simulink model "GS_model"  (R2018b)
settings: Solver=ode5  StartTime=0.0  StopTime=SimuStopTime  FixedStep=T_Simu  RelTol=1e-3
InitFcn:
  | Initial
undefined symbols (not defined in the file or in its folder): Aba10, Aba20, aeroCIP2006_S, aeroCIP2006_X, aeroCIP2006_Y, Agl0, Ass_kS, Ass_n1, Ass_n2, Ass_n3, Ass_n4, Ass_Noise, Ass_R, Ass_Resolution, Ass_TmOrder, AssA_Fix_Abs, AssB_Fix_Abs, AssC_Fix_Abs, AssD_Fix_Abs, AssE_Fix_Aps, AssF_Fix_Aps, C, c_max, c_min, Cd, CenterOfFigNX, CenterOfFigNY, CenterOfFigNZ, CenterOfFigP1, CenterOfFigP2, CenterOfFigPX, CenterOfFigPY, CenterOfFigPZ, Cmu, Crou, DEG2RAD, DiscIntNeverNeededParam, Eg_Dir, Eg_F, Eg_PrepareTime, Eg_r_L_L, Fw_Abf, Fw_Hmax, Fw_J, Fw_Spd0, Fw_Tmax, git_hash_BaseLine, git_hash_Project, Gnss_Noise_Pos, Gnss_Noise_Vel, Gnss_PropgationTime, GyroA_Fix_Abg, GyroA_Noise, GyroB_Fix_Abg, GyroB_Noise, GyroC_Fix_Abg, GyroC_Noise, GyroD_Fix_Abg, GyroD_Noise, h ... (+94)
libraries: simulink x308, sharedutil x46, aerolibutil x37, sharedtransform x31, vrlib x14, aerolibgravity2 x2
(part 9 of 20)

== system GS_model/Subsystem2/Subsystem/Sensor/StA&B&C&DModel1/StAMathModel3/StMathModel ==
  note: Qbs_St
  Qib : Inport
  Cons_StNoise : Inport  Port=2
  Qsb_StFix : Inport  Port=3
  TC_StFixErr : Inport  Port=4
  TC_StNoiseCoff : Inport  Port=5
  StNum : Inport  Port=6
  3 : Subsystem
  Constant : Constant  Value=0
  Constant1 : Constant  Value=0
  Demux : Demux  Outputs=[1;4]
  Demux1 : Demux  Outputs=2
  Logical Operator : Logic  Operator=OR  AllPortsSameDT=off  OutDataTypeStr=boolean
  Logical Operator1 : Logic  Operator=OR  AllPortsSameDT=off  OutDataTypeStr=boolean
  Quaternion Inverse : aerolibutil/Quaternion Inverse
  Quaternion Multiplication : aerolibutil/Quaternion Multiplication
  Quaternion Multiplication2 : aerolibutil/Quaternion Multiplication
  Quaternion Multiplication4 : aerolibutil/Quaternion Multiplication
  Quaternion Normalize : sharedutil/Quaternion Normalize  aMode=aMode
      settings: SourceProductBaseCode=AE,PW,MT,VE,VP
  Quaternion Normalize2 : sharedutil/Quaternion Normalize  aMode=aMode
      settings: SourceProductBaseCode=AE,PW,MT,VE,VP
  Relational Operator{,1..3} (4 alike) : RelationalOperator  Operator===  OutDataTypeStr=boolean  RndMeth=Simplest
  Triggered Subsystem1 : Subsystem  TreatAsAtomicUnit=on
  Triggered Subsystem2 : Subsystem  TreatAsAtomicUnit=on
  Qis_St : Outport
  wires:
  Quaternion Inverse/1 -> Quaternion Multiplication2/2
  Logical Operator1/1 -> Triggered Subsystem2/Enable
  Relational Operator3/1 -> Logical Operator1/1
  Constant1/1 -> Relational Operator3/1
  Relational Operator/1 -> Logical Operator1/2
  Logical Operator/1 -> Triggered Subsystem1/Enable
  Relational Operator2/1 -> Logical Operator/1
  Constant/1 -> Relational Operator2/1
  Relational Operator1/1 -> Logical Operator/2
  StNum/1 -> Relational Operator1/1, Relational Operator/1
  Cons_StNoise/1 -> 3/2(Cons_StNoise)
  Quaternion Multiplication4/1 -> Qis_St/1
  TC_StFixErr/1 -> Demux/1
  Qsb_StFix/1 -> Quaternion Normalize/1
  Qib/1 -> Quaternion Multiplication2/1
  Quaternion Multiplication/1 -> Quaternion Inverse/1
  3/1(Q_StNoise) -> Quaternion Multiplication4/2
  Quaternion Normalize2/1 -> Quaternion Multiplication/2
  TC_StNoiseCoff/1 -> Demux1/1
  Quaternion Multiplication2/1 -> Quaternion Multiplication4/1
  Demux/1 -> Relational Operator1/2, Relational Operator2/2
  Demux1/2 -> Triggered Subsystem2/1(In1)
  Demux1/1 -> Relational Operator/2, Relational Operator3/2
  Quaternion Normalize/1 -> Quaternion Multiplication/1
  Triggered Subsystem1/1(Out1) -> Quaternion Normalize2/1
  Demux/2 -> Triggered Subsystem1/1(In1)
  Triggered Subsystem2/1(Out1) -> 3/1(TC_StNoiseCoff)

== system GS_model/Subsystem2/Subsystem/Sensor/StA&B&C&DModel1/StAMathModel3/Subsystem ==
  note: 0-自主
      | 1-常有效
      | 2-常无效
  Sun_b : Inport
  Sunshine : Inport  Port=2
  Tc_ValidSet : Inport  Port=3
  Qsb_StAFix : Inport  Port=4
  SEA : Inport  Port=5
  EEA : Inport  Port=6
  Qob : Inport  Port=7
  Qis : Inport  Port=8
  StNum : Inport  Port=9
  Constant1 : Constant  Value=0
  Constant2 : Constant  Value=[1;0;0;0]
  Constant3 : Constant
  Constant4 : Constant  Value=0
  Demux1 : Demux  Outputs=2
  Logical Operator1 : Logic  Operator=OR  AllPortsSameDT=off  OutDataTypeStr=boolean
  Relational Operator : RelationalOperator  Operator===  OutDataTypeStr=boolean  RndMeth=Simplest
  Relational Operator3 : RelationalOperator  Operator===  OutDataTypeStr=boolean  RndMeth=Simplest
  Subsystem : Subsystem
  Switch : Switch  Criteria=u2 > Threshold  Threshold=0.5
  Switch1 : Switch  Criteria=u2 > Threshold  Threshold=0.5
  Switch2 : Switch  Criteria=u2 > Threshold  Threshold=1.5
  Triggered Subsystem2 : Subsystem  TreatAsAtomicUnit=on
  Agl_St&SunEarth : Outport
  Valid : Outport  Port=2
  Qis_St : Outport  Port=3
  wires:
  Constant2/1 -> Switch/3
  Qis/1 -> Switch/1
  Logical Operator1/1 -> Triggered Subsystem2/Enable
  Constant4/1 -> Switch2/1
  Switch1/1 -> Switch2/3
  Constant3/1 -> Switch1/1
  Subsystem/1(Valid) -> Switch1/3
  Triggered Subsystem2/1(Out1) -> Switch2/2, Switch1/2
  Tc_ValidSet/1 -> Demux1/1
  Demux1/1 -> Relational Operator/2, Relational Operator3/2
  StNum/1 -> Relational Operator/1
  Demux1/2 -> Triggered Subsystem2/1(In1)
  Constant1/1 -> Relational Operator3/1
  Relational Operator/1 -> Logical Operator1/2
  Relational Operator3/1 -> Logical Operator1/1
  Subsystem/2(Agl_St&SunEarth) -> Agl_St&SunEarth/1
  Qob/1 -> Subsystem/6(Qob)
  EEA/1 -> Subsystem/5(EEA)
  SEA/1 -> Subsystem/4(SEA)
  Qsb_StAFix/1 -> Subsystem/3(Qsb_StAFix)
  Sunshine/1 -> Subsystem/2(Sunshine)
  Sun_b/1 -> Subsystem/1(Sun_b)
  Switch2/1 -> Switch/2, Valid/1
  Switch/1 -> Qis_St/1

== system GS_model/Subsystem2/EquipmentCmd/Fw1/Subsystem7/Subsystem1/FWDataSourceChoice/CmdModeChoice ==
  note: UDP指令来源：复用星上链路标志，默认AA
      | AA -- FC指令
      | 55 -- 直接指令
  note: 动力学链路，默认0
      | 1 -- 422
      | 0 -- UDP
  FW_Data_Source : Inport
  FW_CmdMode : Inport  Port=2
  422 : Subsystem  TreatAsAtomicUnit=on
  Demux : Demux  Outputs=2
  FC : Subsystem  TreatAsAtomicUnit=on
  If : If  NumInputs=2  IfExpression=u1 > 0.5  ElseIfExpressions=u1<0.5 & u2<100
  Merge : Merge  Inputs=3
  Selector : Selector  InputPortWidth=3  IndexOptions=Index vector (dialog)  Indices=1  OutputSizes=1
  Selector1 : Selector  InputPortWidth=3  IndexOptions=Index vector (dialog)  Indices=2  OutputSizes=1
  Selector2 : Selector  InputPortWidth=3  IndexOptions=Index vector (dialog)  Indices=3  OutputSizes=1
  UDP : Subsystem  TreatAsAtomicUnit=on
  FW_Cmd_Mode : Outport
  wires:
  Demux/2 -> If/2
  If/3 -> FC/Action
  If/2 -> UDP/Action
  If/1 -> 422/Action
  FW_Data_Source/1 -> Demux/1
  Demux/1 -> If/1
  Selector2/1 -> FC/1(In1)
  Selector1/1 -> UDP/1(In1)
  Selector/1 -> 422/1(In1)
  Merge/1 -> FW_Cmd_Mode/1
  FC/1(Out1) -> Merge/3
  UDP/1(Out1) -> Merge/2
  422/1(Out1) -> Merge/1
  FW_CmdMode/1 -> Selector/1, Selector1/1, Selector2/1

== system GS_model/Subsystem2/EquipmentCmd/Fw1/Subsystem7/Subsystem1/FWDataSourceChoice/CmdSpdChoice ==
  note: Fc_DataSource      Tc_DataSource
      | AA-真采集（默认）  1-422(DB9);
      |                                  0-反测（默认
      | 55 -伪采集                UDP
  note: AA -- FC
      | 55 -- udp
  note: 1 -- 422
      | 0 -- else
  note: Fc_DataSource
  note: Tc_DataSource
  FW_Data_Source : Inport
  FW_CmdSpd : Inport  Port=2
  422 : Subsystem  TreatAsAtomicUnit=on
  Demux : Demux  Outputs=2
  FC : Subsystem  TreatAsAtomicUnit=on
  If : If  NumInputs=2  IfExpression=u1 > 0.5  ElseIfExpressions=u1<0.5 & u2<100
  Merge : Merge  Inputs=3
  Selector : Selector  InputPortWidth=3  IndexOptions=Index vector (dialog)  Indices=1  OutputSizes=1
  Selector1 : Selector  InputPortWidth=3  IndexOptions=Index vector (dialog)  Indices=2  OutputSizes=1
  Selector2 : Selector  InputPortWidth=3  IndexOptions=Index vector (dialog)  Indices=3  OutputSizes=1
  UDP : Subsystem  TreatAsAtomicUnit=on
  FW_Cmd_Spd : Outport
  wires:
  Demux/2 -> If/2
  If/3 -> FC/Action
  If/2 -> UDP/Action
  If/1 -> 422/Action
  FW_Data_Source/1 -> Demux/1
  Demux/1 -> If/1
  Selector2/1 -> FC/1(In1)
  Selector1/1 -> UDP/1(In1)
  Selector/1 -> 422/1(In1)
  Merge/1 -> FW_Cmd_Spd/1
  FC/1(Out1) -> Merge/3
  UDP/1(Out1) -> Merge/2
  422/1(Out1) -> Merge/1
  FW_CmdSpd/1 -> Selector/1, Selector1/1, Selector2/1

== system GS_model/Subsystem2/EquipmentCmd/Fw1/Subsystem7/Subsystem1/FWDataSourceChoice/CmdTChoice ==
  note: 1 -- 422
      | 0 -- else
  note: AA -- FC
      | 55 -- udp
  FW_Data_Source : Inport
  FW_CmdTorque : Inport  Port=2
  422 : Subsystem  TreatAsAtomicUnit=on
  Demux : Demux  Outputs=2
  FC : Subsystem  TreatAsAtomicUnit=on
  If : If  NumInputs=2  IfExpression=u1 > 0.5  ElseIfExpressions=u1<0.5 & u2<100
  Merge : Merge  Inputs=3
  Selector : Selector  InputPortWidth=3  IndexOptions=Index vector (dialog)  Indices=1  OutputSizes=1
  Selector1 : Selector  InputPortWidth=3  IndexOptions=Index vector (dialog)  Indices=2  OutputSizes=1
  Selector2 : Selector  InputPortWidth=3  IndexOptions=Index vector (dialog)  Indices=3  OutputSizes=1
  UDP : Subsystem  TreatAsAtomicUnit=on
  FW_Cmd_T : Outport
  wires:
  FW_CmdTorque/1 -> Selector2/1, Selector1/1, Selector/1
  422/1(Out1) -> Merge/1
  UDP/1(Out1) -> Merge/2
  FC/1(Out1) -> Merge/3
  Merge/1 -> FW_Cmd_T/1
  Selector/1 -> 422/1(In1)
  Selector1/1 -> UDP/1(In1)
  Selector2/1 -> FC/1(In1)
  Demux/1 -> If/1
  FW_Data_Source/1 -> Demux/1
  If/1 -> 422/Action
  If/2 -> UDP/Action
  If/3 -> FC/Action
  Demux/2 -> If/2

== system GS_model/Subsystem2/EquipmentCmd/Fw1/Subsystem7/Subsystem2/FWDataSourceChoice/CmdModeChoice ==
  note: 动力学链路，默认0
      | 1 -- 422
      | 0 -- UDP
  note: UDP指令来源：复用星上链路标志，默认AA
      | AA -- FC指令
      | 55 -- 直接指令
  FW_Data_Source : Inport
  FW_CmdMode : Inport  Port=2
  422 : Subsystem  TreatAsAtomicUnit=on
  Demux : Demux  Outputs=2
  FC : Subsystem  TreatAsAtomicUnit=on
  If : If  NumInputs=2  IfExpression=u1 > 0.5  ElseIfExpressions=u1<0.5 & u2<100
  Merge : Merge  Inputs=3
  Selector : Selector  InputPortWidth=3  IndexOptions=Index vector (dialog)  Indices=1  OutputSizes=1
  Selector1 : Selector  InputPortWidth=3  IndexOptions=Index vector (dialog)  Indices=2  OutputSizes=1
  Selector2 : Selector  InputPortWidth=3  IndexOptions=Index vector (dialog)  Indices=3  OutputSizes=1
  UDP : Subsystem  TreatAsAtomicUnit=on
  FW_Cmd_Mode : Outport
  wires:
  FW_CmdMode/1 -> Selector2/1, Selector1/1, Selector/1
  422/1(Out1) -> Merge/1
  UDP/1(Out1) -> Merge/2
  FC/1(Out1) -> Merge/3
  Merge/1 -> FW_Cmd_Mode/1
  Selector/1 -> 422/1(In1)
  Selector1/1 -> UDP/1(In1)
  Selector2/1 -> FC/1(In1)
  Demux/1 -> If/1
  FW_Data_Source/1 -> Demux/1
  If/1 -> 422/Action
  If/2 -> UDP/Action
  If/3 -> FC/Action
  Demux/2 -> If/2

== system GS_model/Subsystem2/EquipmentCmd/Fw1/Subsystem7/Subsystem2/FWDataSourceChoice/CmdSpdChoice ==
  note: Tc_DataSource
  note: Fc_DataSource
  note: 1 -- 422
      | 0 -- else
  note: AA -- FC
      | 55 -- udp
  note: Fc_DataSource      Tc_DataSource
      | AA-真采集（默认）  1-422(DB9);
      |                                  0-反测（默认
      | 55 -伪采集                UDP
  FW_Data_Source : Inport
  FW_CmdSpd : Inport  Port=2
  422 : Subsystem  TreatAsAtomicUnit=on
  Demux : Demux  Outputs=2
  FC : Subsystem  TreatAsAtomicUnit=on
  If : If  NumInputs=2  IfExpression=u1 > 0.5  ElseIfExpressions=u1<0.5 & u2<100
  Merge : Merge  Inputs=3
  Selector : Selector  InputPortWidth=3  IndexOptions=Index vector (dialog)  Indices=1  OutputSizes=1
  Selector1 : Selector  InputPortWidth=3  IndexOptions=Index vector (dialog)  Indices=2  OutputSizes=1
  Selector2 : Selector  InputPortWidth=3  IndexOptions=Index vector (dialog)  Indices=3  OutputSizes=1
  UDP : Subsystem  TreatAsAtomicUnit=on
  FW_Cmd_Spd : Outport
  wires:
  FW_CmdSpd/1 -> Selector2/1, Selector1/1, Selector/1
  422/1(Out1) -> Merge/1
  UDP/1(Out1) -> Merge/2
  FC/1(Out1) -> Merge/3
  Merge/1 -> FW_Cmd_Spd/1
  Selector/1 -> 422/1(In1)
  Selector1/1 -> UDP/1(In1)
  Selector2/1 -> FC/1(In1)
  Demux/1 -> If/1
  FW_Data_Source/1 -> Demux/1
  If/1 -> 422/Action
  If/2 -> UDP/Action
  If/3 -> FC/Action
  Demux/2 -> If/2

== system GS_model/Subsystem2/EquipmentCmd/Fw1/Subsystem7/Subsystem2/FWDataSourceChoice/CmdTChoice ==
  note: AA -- FC
      | 55 -- udp
  note: 1 -- 422
      | 0 -- else
  FW_Data_Source : Inport
  FW_CmdTorque : Inport  Port=2
  422 : Subsystem  TreatAsAtomicUnit=on
  Demux : Demux  Outputs=2
  FC : Subsystem  TreatAsAtomicUnit=on
  If : If  NumInputs=2  IfExpression=u1 > 0.5  ElseIfExpressions=u1<0.5 & u2<100
  Merge : Merge  Inputs=3
  Selector : Selector  InputPortWidth=3  IndexOptions=Index vector (dialog)  Indices=1  OutputSizes=1
  Selector1 : Selector  InputPortWidth=3  IndexOptions=Index vector (dialog)  Indices=2  OutputSizes=1
  Selector2 : Selector  InputPortWidth=3  IndexOptions=Index vector (dialog)  Indices=3  OutputSizes=1
  UDP : Subsystem  TreatAsAtomicUnit=on
  FW_Cmd_T : Outport
  wires:
  Demux/2 -> If/2
  If/3 -> FC/Action
  If/2 -> UDP/Action
  If/1 -> 422/Action
  FW_Data_Source/1 -> Demux/1
  Demux/1 -> If/1
  Selector2/1 -> FC/1(In1)
  Selector1/1 -> UDP/1(In1)
  Selector/1 -> 422/1(In1)
  Merge/1 -> FW_Cmd_T/1
  FC/1(Out1) -> Merge/3
  UDP/1(Out1) -> Merge/2
  422/1(Out1) -> Merge/1
  FW_CmdTorque/1 -> Selector/1, Selector1/1, Selector2/1

== system GS_model/Subsystem2/EquipmentCmd/Fw1/Subsystem7/Subsystem3/FWDataSourceChoice/CmdModeChoice ==
  note: UDP指令来源：复用星上链路标志，默认AA
      | AA -- FC指令
      | 55 -- 直接指令
  note: 动力学链路，默认0
      | 1 -- 422
      | 0 -- UDP
  FW_Data_Source : Inport
  FW_CmdMode : Inport  Port=2
  422 : Subsystem  TreatAsAtomicUnit=on
  Demux : Demux  Outputs=2
  FC : Subsystem  TreatAsAtomicUnit=on
  If : If  NumInputs=2  IfExpression=u1 > 0.5  ElseIfExpressions=u1<0.5 & u2<100
  Merge : Merge  Inputs=3
  Selector : Selector  InputPortWidth=3  IndexOptions=Index vector (dialog)  Indices=1  OutputSizes=1
  Selector1 : Selector  InputPortWidth=3  IndexOptions=Index vector (dialog)  Indices=2  OutputSizes=1
  Selector2 : Selector  InputPortWidth=3  IndexOptions=Index vector (dialog)  Indices=3  OutputSizes=1
  UDP : Subsystem  TreatAsAtomicUnit=on
  FW_Cmd_Mode : Outport
  wires:
  Demux/2 -> If/2
  If/3 -> FC/Action
  If/2 -> UDP/Action
  If/1 -> 422/Action
  FW_Data_Source/1 -> Demux/1
  Demux/1 -> If/1
  Selector2/1 -> FC/1(In1)
  Selector1/1 -> UDP/1(In1)
  Selector/1 -> 422/1(In1)
  Merge/1 -> FW_Cmd_Mode/1
  FC/1(Out1) -> Merge/3
  UDP/1(Out1) -> Merge/2
  422/1(Out1) -> Merge/1
  FW_CmdMode/1 -> Selector/1, Selector1/1, Selector2/1

== system GS_model/Subsystem2/EquipmentCmd/Fw1/Subsystem7/Subsystem3/FWDataSourceChoice/CmdSpdChoice ==
  note: Fc_DataSource      Tc_DataSource
      | AA-真采集（默认）  1-422(DB9);
      |                                  0-反测（默认
      | 55 -伪采集                UDP
  note: AA -- FC
      | 55 -- udp
  note: 1 -- 422
      | 0 -- else
  note: Fc_DataSource
  note: Tc_DataSource
  FW_Data_Source : Inport
  FW_CmdSpd : Inport  Port=2
  422 : Subsystem  TreatAsAtomicUnit=on
  Demux : Demux  Outputs=2
  FC : Subsystem  TreatAsAtomicUnit=on
  If : If  NumInputs=2  IfExpression=u1 > 0.5  ElseIfExpressions=u1<0.5 & u2<100
  Merge : Merge  Inputs=3
  Selector : Selector  InputPortWidth=3  IndexOptions=Index vector (dialog)  Indices=1  OutputSizes=1
  Selector1 : Selector  InputPortWidth=3  IndexOptions=Index vector (dialog)  Indices=2  OutputSizes=1
  Selector2 : Selector  InputPortWidth=3  IndexOptions=Index vector (dialog)  Indices=3  OutputSizes=1
  UDP : Subsystem  TreatAsAtomicUnit=on
  FW_Cmd_Spd : Outport
  wires:
  Demux/2 -> If/2
  If/3 -> FC/Action
  If/2 -> UDP/Action
  If/1 -> 422/Action
  FW_Data_Source/1 -> Demux/1
  Demux/1 -> If/1
  Selector2/1 -> FC/1(In1)
  Selector1/1 -> UDP/1(In1)
  Selector/1 -> 422/1(In1)
  Merge/1 -> FW_Cmd_Spd/1
  FC/1(Out1) -> Merge/3
  UDP/1(Out1) -> Merge/2
  422/1(Out1) -> Merge/1
  FW_CmdSpd/1 -> Selector/1, Selector1/1, Selector2/1

== system GS_model/Subsystem2/EquipmentCmd/Fw1/Subsystem7/Subsystem3/FWDataSourceChoice/CmdTChoice ==
  note: 1 -- 422
      | 0 -- else
  note: AA -- FC
      | 55 -- udp
  FW_Data_Source : Inport
  FW_CmdTorque : Inport  Port=2
  422 : Subsystem  TreatAsAtomicUnit=on
  Demux : Demux  Outputs=2
  FC : Subsystem  TreatAsAtomicUnit=on
  If : If  NumInputs=2  IfExpression=u1 > 0.5  ElseIfExpressions=u1<0.5 & u2<100
  Merge : Merge  Inputs=3
  Selector : Selector  InputPortWidth=3  IndexOptions=Index vector (dialog)  Indices=1  OutputSizes=1
  Selector1 : Selector  InputPortWidth=3  IndexOptions=Index vector (dialog)  Indices=2  OutputSizes=1
  Selector2 : Selector  InputPortWidth=3  IndexOptions=Index vector (dialog)  Indices=3  OutputSizes=1
  UDP : Subsystem  TreatAsAtomicUnit=on
  FW_Cmd_T : Outport
  wires:
  FW_CmdTorque/1 -> Selector2/1, Selector1/1, Selector/1
  422/1(Out1) -> Merge/1
  UDP/1(Out1) -> Merge/2
  FC/1(Out1) -> Merge/3
  Merge/1 -> FW_Cmd_T/1
  Selector/1 -> 422/1(In1)
  Selector1/1 -> UDP/1(In1)
  Selector2/1 -> FC/1(In1)
  Demux/1 -> If/1
  FW_Data_Source/1 -> Demux/1
  If/1 -> 422/Action
  If/2 -> UDP/Action
  If/3 -> FC/Action
  Demux/2 -> If/2

== system GS_model/Subsystem2/EquipmentCmd/Fw1/Subsystem7/Subsystem4/FWDataSourceChoice/CmdModeChoice ==
  note: 动力学链路，默认0
      | 1 -- 422
      | 0 -- UDP
  note: UDP指令来源：复用星上链路标志，默认AA
      | AA -- FC指令
      | 55 -- 直接指令
  FW_Data_Source : Inport
  FW_CmdMode : Inport  Port=2
  422 : Subsystem  TreatAsAtomicUnit=on
  Demux : Demux  Outputs=2
  FC : Subsystem  TreatAsAtomicUnit=on
  If : If  NumInputs=2  IfExpression=u1 > 0.5  ElseIfExpressions=u1<0.5 & u2<100
  Merge : Merge  Inputs=3
  Selector : Selector  InputPortWidth=3  IndexOptions=Index vector (dialog)  Indices=1  OutputSizes=1
  Selector1 : Selector  InputPortWidth=3  IndexOptions=Index vector (dialog)  Indices=2  OutputSizes=1
  Selector2 : Selector  InputPortWidth=3  IndexOptions=Index vector (dialog)  Indices=3  OutputSizes=1
  UDP : Subsystem  TreatAsAtomicUnit=on
  FW_Cmd_Mode : Outport
  wires:
  FW_CmdMode/1 -> Selector2/1, Selector1/1, Selector/1
  422/1(Out1) -> Merge/1
  UDP/1(Out1) -> Merge/2
  FC/1(Out1) -> Merge/3
  Merge/1 -> FW_Cmd_Mode/1
  Selector/1 -> 422/1(In1)
  Selector1/1 -> UDP/1(In1)
  Selector2/1 -> FC/1(In1)
  Demux/1 -> If/1
  FW_Data_Source/1 -> Demux/1
  If/1 -> 422/Action
  If/2 -> UDP/Action
  If/3 -> FC/Action
  Demux/2 -> If/2

== system GS_model/Subsystem2/EquipmentCmd/Fw1/Subsystem7/Subsystem4/FWDataSourceChoice/CmdSpdChoice ==
  note: Tc_DataSource
  note: Fc_DataSource
  note: 1 -- 422
      | 0 -- else
  note: AA -- FC
      | 55 -- udp
  note: Fc_DataSource      Tc_DataSource
      | AA-真采集（默认）  1-422(DB9);
      |                                  0-反测（默认
      | 55 -伪采集                UDP
  FW_Data_Source : Inport
  FW_CmdSpd : Inport  Port=2
  422 : Subsystem  TreatAsAtomicUnit=on
  Demux : Demux  Outputs=2
  FC : Subsystem  TreatAsAtomicUnit=on
  If : If  NumInputs=2  IfExpression=u1 > 0.5  ElseIfExpressions=u1<0.5 & u2<100
  Merge : Merge  Inputs=3
  Selector : Selector  InputPortWidth=3  IndexOptions=Index vector (dialog)  Indices=1  OutputSizes=1
  Selector1 : Selector  InputPortWidth=3  IndexOptions=Index vector (dialog)  Indices=2  OutputSizes=1
  Selector2 : Selector  InputPortWidth=3  IndexOptions=Index vector (dialog)  Indices=3  OutputSizes=1
  UDP : Subsystem  TreatAsAtomicUnit=on
  FW_Cmd_Spd : Outport
  wires:
  FW_CmdSpd/1 -> Selector2/1, Selector1/1, Selector/1
  422/1(Out1) -> Merge/1
  UDP/1(Out1) -> Merge/2
  FC/1(Out1) -> Merge/3
  Merge/1 -> FW_Cmd_Spd/1
  Selector/1 -> 422/1(In1)
  Selector1/1 -> UDP/1(In1)
  Selector2/1 -> FC/1(In1)
  Demux/1 -> If/1
  FW_Data_Source/1 -> Demux/1
  If/1 -> 422/Action
  If/2 -> UDP/Action
  If/3 -> FC/Action
  Demux/2 -> If/2

== system GS_model/Subsystem2/EquipmentCmd/Fw1/Subsystem7/Subsystem4/FWDataSourceChoice/CmdTChoice ==
  note: AA -- FC
      | 55 -- udp
  note: 1 -- 422
      | 0 -- else
  FW_Data_Source : Inport
  FW_CmdTorque : Inport  Port=2
  422 : Subsystem  TreatAsAtomicUnit=on
  Demux : Demux  Outputs=2
  FC : Subsystem  TreatAsAtomicUnit=on
  If : If  NumInputs=2  IfExpression=u1 > 0.5  ElseIfExpressions=u1<0.5 & u2<100
  Merge : Merge  Inputs=3
  Selector : Selector  InputPortWidth=3  IndexOptions=Index vector (dialog)  Indices=1  OutputSizes=1
  Selector1 : Selector  InputPortWidth=3  IndexOptions=Index vector (dialog)  Indices=2  OutputSizes=1
  Selector2 : Selector  InputPortWidth=3  IndexOptions=Index vector (dialog)  Indices=3  OutputSizes=1
  UDP : Subsystem  TreatAsAtomicUnit=on
  FW_Cmd_T : Outport
  wires:
  Demux/2 -> If/2
  If/3 -> FC/Action
  If/2 -> UDP/Action
  If/1 -> 422/Action
  FW_Data_Source/1 -> Demux/1
  Demux/1 -> If/1
  Selector2/1 -> FC/1(In1)
  Selector1/1 -> UDP/1(In1)
  Selector/1 -> 422/1(In1)
  Merge/1 -> FW_Cmd_T/1
  FC/1(Out1) -> Merge/3
  UDP/1(Out1) -> Merge/2
  422/1(Out1) -> Merge/1
  FW_CmdTorque/1 -> Selector/1, Selector1/1, Selector2/1

== system GS_model/Subsystem2/EquipmentCmd/Fw1/Subsystem7/Subsystem5/FWDataSourceChoice/CmdModeChoice ==
  note: UDP指令来源：复用星上链路标志，默认AA
      | AA -- FC指令
      | 55 -- 直接指令
  note: 动力学链路，默认0
      | 1 -- 422
      | 0 -- UDP
  FW_Data_Source : Inport
  FW_CmdMode : Inport  Port=2
  422 : Subsystem  TreatAsAtomicUnit=on
  Demux : Demux  Outputs=2
  FC : Subsystem  TreatAsAtomicUnit=on
  If : If  NumInputs=2  IfExpression=u1 > 0.5  ElseIfExpressions=u1<0.5 & u2<100
  Merge : Merge  Inputs=3
  Selector : Selector  InputPortWidth=3  IndexOptions=Index vector (dialog)  Indices=1  OutputSizes=1
  Selector1 : Selector  InputPortWidth=3  IndexOptions=Index vector (dialog)  Indices=2  OutputSizes=1
  Selector2 : Selector  InputPortWidth=3  IndexOptions=Index vector (dialog)  Indices=3  OutputSizes=1
  UDP : Subsystem  TreatAsAtomicUnit=on
  FW_Cmd_Mode : Outport
  wires:
  Demux/2 -> If/2
  If/3 -> FC/Action
  If/2 -> UDP/Action
  If/1 -> 422/Action
  FW_Data_Source/1 -> Demux/1
  Demux/1 -> If/1
  Selector2/1 -> FC/1(In1)
  Selector1/1 -> UDP/1(In1)
  Selector/1 -> 422/1(In1)
  Merge/1 -> FW_Cmd_Mode/1
  FC/1(Out1) -> Merge/3
  UDP/1(Out1) -> Merge/2
  422/1(Out1) -> Merge/1
  FW_CmdMode/1 -> Selector/1, Selector1/1, Selector2/1

== system GS_model/Subsystem2/EquipmentCmd/Fw1/Subsystem7/Subsystem5/FWDataSourceChoice/CmdSpdChoice ==
  note: Fc_DataSource      Tc_DataSource
      | AA-真采集（默认）  1-422(DB9);
      |                                  0-反测（默认
      | 55 -伪采集                UDP
  note: AA -- FC
      | 55 -- udp
  note: 1 -- 422
      | 0 -- else
  note: Fc_DataSource
  note: Tc_DataSource
  FW_Data_Source : Inport
  FW_CmdSpd : Inport  Port=2
  422 : Subsystem  TreatAsAtomicUnit=on
  Demux : Demux  Outputs=2
  FC : Subsystem  TreatAsAtomicUnit=on
  If : If  NumInputs=2  IfExpression=u1 > 0.5  ElseIfExpressions=u1<0.5 & u2<100
  Merge : Merge  Inputs=3
  Selector : Selector  InputPortWidth=3  IndexOptions=Index vector (dialog)  Indices=1  OutputSizes=1
  Selector1 : Selector  InputPortWidth=3  IndexOptions=Index vector (dialog)  Indices=2  OutputSizes=1
  Selector2 : Selector  InputPortWidth=3  IndexOptions=Index vector (dialog)  Indices=3  OutputSizes=1
  UDP : Subsystem  TreatAsAtomicUnit=on
  FW_Cmd_Spd : Outport
  wires:
  Demux/2 -> If/2
  If/3 -> FC/Action
  If/2 -> UDP/Action
  If/1 -> 422/Action
  FW_Data_Source/1 -> Demux/1
  Demux/1 -> If/1
  Selector2/1 -> FC/1(In1)
  Selector1/1 -> UDP/1(In1)
  Selector/1 -> 422/1(In1)
  Merge/1 -> FW_Cmd_Spd/1
  FC/1(Out1) -> Merge/3
  UDP/1(Out1) -> Merge/2
  422/1(Out1) -> Merge/1
  FW_CmdSpd/1 -> Selector/1, Selector1/1, Selector2/1

== system GS_model/Subsystem2/EquipmentCmd/Fw1/Subsystem7/Subsystem5/FWDataSourceChoice/CmdTChoice ==
  note: 1 -- 422
      | 0 -- else
  note: AA -- FC
      | 55 -- udp
  FW_Data_Source : Inport
  FW_CmdTorque : Inport  Port=2
  422 : Subsystem  TreatAsAtomicUnit=on
  Demux : Demux  Outputs=2
  FC : Subsystem  TreatAsAtomicUnit=on
  If : If  NumInputs=2  IfExpression=u1 > 0.5  ElseIfExpressions=u1<0.5 & u2<100
  Merge : Merge  Inputs=3
  Selector : Selector  InputPortWidth=3  IndexOptions=Index vector (dialog)  Indices=1  OutputSizes=1
  Selector1 : Selector  InputPortWidth=3  IndexOptions=Index vector (dialog)  Indices=2  OutputSizes=1
  Selector2 : Selector  InputPortWidth=3  IndexOptions=Index vector (dialog)  Indices=3  OutputSizes=1
  UDP : Subsystem  TreatAsAtomicUnit=on
  FW_Cmd_T : Outport
  wires:
  FW_CmdTorque/1 -> Selector2/1, Selector1/1, Selector/1
  422/1(Out1) -> Merge/1
  UDP/1(Out1) -> Merge/2
  FC/1(Out1) -> Merge/3
  Merge/1 -> FW_Cmd_T/1
  Selector/1 -> 422/1(In1)
  Selector1/1 -> UDP/1(In1)
  Selector2/1 -> FC/1(In1)
  Demux/1 -> If/1
  FW_Data_Source/1 -> Demux/1
  If/1 -> 422/Action
  If/2 -> UDP/Action
  If/3 -> FC/Action
  Demux/2 -> If/2

== system GS_model/Subsystem2/EquipmentCmd/Fw1/Subsystem7/Subsystem6/FWDataSourceChoice/CmdModeChoice ==
  note: 动力学链路，默认0
      | 1 -- 422
      | 0 -- UDP
  note: UDP指令来源：复用星上链路标志，默认AA
      | AA -- FC指令
      | 55 -- 直接指令
  FW_Data_Source : Inport
  FW_CmdMode : Inport  Port=2
  422 : Subsystem  TreatAsAtomicUnit=on
  Demux : Demux  Outputs=2
  FC : Subsystem  TreatAsAtomicUnit=on
  If : If  NumInputs=2  IfExpression=u1 > 0.5  ElseIfExpressions=u1<0.5 & u2<100
  Merge : Merge  Inputs=3
  Selector : Selector  InputPortWidth=3  IndexOptions=Index vector (dialog)  Indices=1  OutputSizes=1
  Selector1 : Selector  InputPortWidth=3  IndexOptions=Index vector (dialog)  Indices=2  OutputSizes=1
  Selector2 : Selector  InputPortWidth=3  IndexOptions=Index vector (dialog)  Indices=3  OutputSizes=1
  UDP : Subsystem  TreatAsAtomicUnit=on
  FW_Cmd_Mode : Outport
  wires:
  FW_CmdMode/1 -> Selector2/1, Selector1/1, Selector/1
  422/1(Out1) -> Merge/1
  UDP/1(Out1) -> Merge/2
  FC/1(Out1) -> Merge/3
  Merge/1 -> FW_Cmd_Mode/1
  Selector/1 -> 422/1(In1)
  Selector1/1 -> UDP/1(In1)
  Selector2/1 -> FC/1(In1)
  Demux/1 -> If/1
  FW_Data_Source/1 -> Demux/1
  If/1 -> 422/Action
  If/2 -> UDP/Action
  If/3 -> FC/Action
  Demux/2 -> If/2

== system GS_model/Subsystem2/EquipmentCmd/Fw1/Subsystem7/Subsystem6/FWDataSourceChoice/CmdSpdChoice ==
  note: Tc_DataSource
  note: Fc_DataSource
  note: 1 -- 422
      | 0 -- else
  note: AA -- FC
      | 55 -- udp
  note: Fc_DataSource      Tc_DataSource
      | AA-真采集（默认）  1-422(DB9);
      |                                  0-反测（默认
      | 55 -伪采集                UDP
  FW_Data_Source : Inport
  FW_CmdSpd : Inport  Port=2
  422 : Subsystem  TreatAsAtomicUnit=on
  Demux : Demux  Outputs=2
  FC : Subsystem  TreatAsAtomicUnit=on
  If : If  NumInputs=2  IfExpression=u1 > 0.5  ElseIfExpressions=u1<0.5 & u2<100
  Merge : Merge  Inputs=3
  Selector : Selector  InputPortWidth=3  IndexOptions=Index vector (dialog)  Indices=1  OutputSizes=1
  Selector1 : Selector  InputPortWidth=3  IndexOptions=Index vector (dialog)  Indices=2  OutputSizes=1
  Selector2 : Selector  InputPortWidth=3  IndexOptions=Index vector (dialog)  Indices=3  OutputSizes=1
  UDP : Subsystem  TreatAsAtomicUnit=on
  FW_Cmd_Spd : Outport
  wires:
  FW_CmdSpd/1 -> Selector2/1, Selector1/1, Selector/1
  422/1(Out1) -> Merge/1
  UDP/1(Out1) -> Merge/2
  FC/1(Out1) -> Merge/3
  Merge/1 -> FW_Cmd_Spd/1
  Selector/1 -> 422/1(In1)
  Selector1/1 -> UDP/1(In1)
  Selector2/1 -> FC/1(In1)
  Demux/1 -> If/1
  FW_Data_Source/1 -> Demux/1
  If/1 -> 422/Action
  If/2 -> UDP/Action
  If/3 -> FC/Action
  Demux/2 -> If/2

== system GS_model/Subsystem2/EquipmentCmd/Fw1/Subsystem7/Subsystem6/FWDataSourceChoice/CmdTChoice ==
  note: AA -- FC
      | 55 -- udp
  note: 1 -- 422
      | 0 -- else
  FW_Data_Source : Inport
  FW_CmdTorque : Inport  Port=2
  422 : Subsystem  TreatAsAtomicUnit=on
  Demux : Demux  Outputs=2
  FC : Subsystem  TreatAsAtomicUnit=on
  If : If  NumInputs=2  IfExpression=u1 > 0.5  ElseIfExpressions=u1<0.5 & u2<100
  Merge : Merge  Inputs=3
  Selector : Selector  InputPortWidth=3  IndexOptions=Index vector (dialog)  Indices=1  OutputSizes=1
  Selector1 : Selector  InputPortWidth=3  IndexOptions=Index vector (dialog)  Indices=2  OutputSizes=1
  Selector2 : Selector  InputPortWidth=3  IndexOptions=Index vector (dialog)  Indices=3  OutputSizes=1
  UDP : Subsystem  TreatAsAtomicUnit=on
  FW_Cmd_T : Outport
  wires:
  Demux/2 -> If/2
  If/3 -> FC/Action
  If/2 -> UDP/Action
  If/1 -> 422/Action
  FW_Data_Source/1 -> Demux/1
  Demux/1 -> If/1
  Selector2/1 -> FC/1(In1)
  Selector1/1 -> UDP/1(In1)
  Selector/1 -> 422/1(In1)
  Merge/1 -> FW_Cmd_T/1
  FC/1(Out1) -> Merge/3
  UDP/1(Out1) -> Merge/2
  422/1(Out1) -> Merge/1
  FW_CmdTorque/1 -> Selector/1, Selector1/1, Selector2/1

== system GS_model/Subsystem2/Subsystem/Actuator/Engine/Subsystem/Subsystem/Triggered Subsystem1 ==
  In1 : Inport
  Enable : EnablePort
  Out1 : Outport  InitialOutput=0
  wires:
  In1/1 -> Out1/1

== system GS_model/Subsystem2/Subsystem/Actuator/Engine/Subsystem/Subsystem1/Triggered Subsystem1 ==
  In1 : Inport
  Enable : EnablePort
  Out1 : Outport  InitialOutput=0
  wires:
  In1/1 -> Out1/1

== system GS_model/Subsystem2/Subsystem/Actuator/Engine/Subsystem/Subsystem2/Triggered Subsystem1 ==
  In1 : Inport
  Enable : EnablePort
  Out1 : Outport  InitialOutput=0
  wires:
  In1/1 -> Out1/1

== system GS_model/Subsystem2/Subsystem/Actuator/Engine/Subsystem1/Subsystem/Triggered Subsystem1 ==
  In1 : Inport
  Enable : EnablePort
  Out1 : Outport  InitialOutput=0
  wires:
  In1/1 -> Out1/1

== system GS_model/Subsystem2/Subsystem/Actuator/Engine/Subsystem1/Subsystem1/Triggered Subsystem1 ==
  In1 : Inport
  Enable : EnablePort
  Out1 : Outport  InitialOutput=0
  wires:
  In1/1 -> Out1/1

== system GS_model/Subsystem2/Subsystem/Actuator/Engine/Subsystem1/Subsystem2/Triggered Subsystem1 ==
  In1 : Inport
  Enable : EnablePort
  Out1 : Outport  InitialOutput=0
  wires:
  In1/1 -> Out1/1

== system GS_model/Subsystem2/Subsystem/Actuator/FlyWheel/FwAModel1/FWDataSourceChoice/DelayModel ==
  TC_FW_Delay : Inport
  FW_Cmd_Mode : Inport  Port=2
  FW_Cmd_Spd : Inport  Port=3
  FW_Cmd_T : Inport  Port=4
  Constant3 : Constant
  Sum8 : Sum  Inputs=|++
  delay1 : Subsystem
  delay2 : Subsystem
  delay3 : Subsystem
  Cmd_Mode : Outport
  Cmd_Spd : Outport  Port=2
  Cmd_T : Outport  Port=3
  wires:
  delay2/1(Out1) -> Cmd_T/1
  FW_Cmd_T/1 -> delay2/2(In2)
  delay1/1(Out1) -> Cmd_Spd/1
  Sum8/1 -> delay1/1(In1), delay2/1(In1), delay3/1(In1)
  FW_Cmd_Spd/1 -> delay1/2(In2)
  Constant3/1 -> Sum8/2
  TC_FW_Delay/1 -> Sum8/1
  FW_Cmd_Mode/1 -> delay3/2(In2)
  delay3/1(Out1) -> Cmd_Mode/1

== system GS_model/Subsystem2/Subsystem/Actuator/FlyWheel/FwAModel1/FWMath&ErrModel/Subsystem1 ==
  Fb_FW_T : Inport
  TC_FW_TSet : Inport  Port=2
  FWNum : Inport  Port=3
  TC_FWErr_TOp : Inport  Port=4
  Compare To Constant : simulink/Logic and Bit Operations/Compare To Constant  relop===  const=0  OutDataTypeStr=boolean
  Compare To Constant1 : simulink/Logic and Bit Operations/Compare To Constant  relop===  const=0  OutDataTypeStr=boolean
  Demux : Demux  Outputs=[1;2]
  Demux1 : Demux  Outputs=2
  Demux2 : Demux  Outputs=2
  If : If  IfExpression=u1 == 1
  If Action Subsystem : Subsystem  TreatAsAtomicUnit=on
  If Action Subsystem1 : Subsystem  TreatAsAtomicUnit=on
  Logical Operator : Logic  Operator=OR  AllPortsSameDT=off  OutDataTypeStr=boolean
  Logical Operator1 : Logic  Operator=OR  AllPortsSameDT=off  OutDataTypeStr=boolean
  Merge : Merge
  Relational Operator1 : RelationalOperator  Operator===  OutDataTypeStr=boolean  RndMeth=Simplest
  Relational Operator3 : RelationalOperator  Operator===  OutDataTypeStr=boolean  RndMeth=Simplest
  Sum : Sum  Inputs=|++
  Triggered Subsystem1 : Subsystem  TreatAsAtomicUnit=on
      mask Display: disp('FWChoice')
  Triggered Subsystem2 : Subsystem  TreatAsAtomicUnit=on
      mask Display: disp('FWChoice')
  TM_FW_T : Outport
  wires:
  Fb_FW_T/1 -> Sum/2
  If/2 -> If Action Subsystem1/Action
  Demux1/2 -> If Action Subsystem/1(In1)
  If Action Subsystem1/1(Out1) -> Merge/2
  Triggered Subsystem2/1(Out1) -> Sum/1
  Demux2/2 -> Triggered Subsystem2/1(In1)
  TC_FWErr_TOp/1 -> Demux2/1
  Merge/1 -> TM_FW_T/1
  Sum/1 -> If Action Subsystem1/1(In1)
  TC_FW_TSet/1 -> Demux/1
  If/1 -> If Action Subsystem/Action
  Demux/2 -> Triggered Subsystem1/1(In1)
  Triggered Subsystem1/1(Out1) -> Demux1/1
  If Action Subsystem/1(Out1) -> Merge/1
  Demux1/1 -> If/1
  Compare To Constant/1 -> Logical Operator/1
  Relational Operator3/1 -> Logical Operator/2
  Demux/1 -> Compare To Constant/1, Relational Operator3/2
  Logical Operator/1 -> Triggered Subsystem1/Enable
  Logical Operator1/1 -> Triggered Subsystem2/Enable
  Demux2/1 -> Relational Operator1/2, Compare To Constant1/1
  Relational Operator1/1 -> Logical Operator1/2
  Compare To Constant1/1 -> Logical Operator1/1
  FWNum/1 -> Relational Operator1/1, Relational Operator3/1

== system GS_model/Subsystem2/Subsystem/Actuator/FlyWheel/FwAModel1/FWMath&ErrModel/Subsystem2 ==
  Fb_FW_Spd : Inport
  TC_FW_SpdSet : Inport  Port=2
  FWNum : Inport  Port=3
  TC_FWErr_SpdOp : Inport  Port=4
  Compare To Constant : simulink/Logic and Bit Operations/Compare To Constant  relop===  const=0  OutDataTypeStr=boolean
  Compare To Constant1 : simulink/Logic and Bit Operations/Compare To Constant  relop===  const=0  OutDataTypeStr=boolean
  Demux : Demux  Outputs=[1;2]
  Demux1 : Demux  Outputs=2
  Demux2 : Demux  Outputs=2
  If : If  IfExpression=u1 == 1
  If Action Subsystem : Subsystem  TreatAsAtomicUnit=on
  If Action Subsystem1 : Subsystem  TreatAsAtomicUnit=on
  Logical Operator : Logic  Operator=OR  AllPortsSameDT=off  OutDataTypeStr=boolean
  Logical Operator1 : Logic  Operator=OR  AllPortsSameDT=off  OutDataTypeStr=boolean
  Merge : Merge
  Relational Operator1 : RelationalOperator  Operator===  OutDataTypeStr=boolean  RndMeth=Simplest
  Relational Operator2 : RelationalOperator  Operator===  OutDataTypeStr=boolean  RndMeth=Simplest
  Sum : Sum  Inputs=|++
  Triggered Subsystem1 : Subsystem  TreatAsAtomicUnit=on
      mask Display: disp('FWChoice')
  Triggered Subsystem2 : Subsystem  TreatAsAtomicUnit=on
      mask Display: disp('FWChoice')
  TM_FW_Spd : Outport
  wires:
  TC_FW_SpdSet/1 -> Demux/1
  Demux/1 -> Compare To Constant/1, Relational Operator1/2
  Merge/1 -> TM_FW_Spd/1
  If/1 -> If Action Subsystem/Action
  TC_FWErr_SpdOp/1 -> Demux2/1
  Triggered Subsystem2/1(Out1) -> Sum/1
  Sum/1 -> If Action Subsystem1/1(In1)
  Demux1/2 -> If Action Subsystem/1(In1)
  Demux2/2 -> Triggered Subsystem2/1(In1)
  Demux1/1 -> If/1
  If Action Subsystem1/1(Out1) -> Merge/2
  Demux/2 -> Triggered Subsystem1/1(In1)
  Fb_FW_Spd/1 -> Sum/2
  Triggered Subsystem1/1(Out1) -> Demux1/1
  FWNum/1 -> Relational Operator2/1, Relational Operator1/1
  Demux2/1 -> Compare To Constant1/1, Relational Operator2/2
  If Action Subsystem/1(Out1) -> Merge/1
  If/2 -> If Action Subsystem1/Action
  Relational Operator1/1 -> Logical Operator/2
  Compare To Constant/1 -> Logical Operator/1
  Logical Operator/1 -> Triggered Subsystem1/Enable
  Relational Operator2/1 -> Logical Operator1/2
  Compare To Constant1/1 -> Logical Operator1/1
  Logical Operator1/1 -> Triggered Subsystem2/Enable

== system GS_model/Subsystem2/Subsystem/Actuator/FlyWheel/FwAModel1/FWMath&ErrModel/Subsystem4 ==
  FWNum : Inport
  FW_Mode : Inport  Port=2
  TC_FW_ModeSet : Inport  Port=3
  Compare To Constant : simulink/Logic and Bit Operations/Compare To Constant  relop===  const=0  OutDataTypeStr=boolean
  Demux : Demux  Outputs=[1;2]
  Demux1 : Demux  Outputs=2
  If : If  IfExpression=u1 == 1
  If Action Subsystem : Subsystem  TreatAsAtomicUnit=on
  If Action Subsystem1 : Subsystem  TreatAsAtomicUnit=on
  Logical Operator : Logic  Operator=OR  AllPortsSameDT=off  OutDataTypeStr=boolean
  Merge : Merge
  Relational Operator1 : RelationalOperator  Operator===  OutDataTypeStr=boolean  RndMeth=Simplest
  Triggered Subsystem1 : Subsystem  TreatAsAtomicUnit=on
      mask Display: disp('FWChoice')
  Fb_FW_Mode : Outport
  wires:
  Merge/1 -> Fb_FW_Mode/1
  If Action Subsystem1/1(Out1) -> Merge/2
  If Action Subsystem/1(Out1) -> Merge/1
  FW_Mode/1 -> If Action Subsystem1/1(In1)
  If/2 -> If Action Subsystem1/Action
  Triggered Subsystem1/1(Out1) -> Demux1/1
  Demux1/2 -> If Action Subsystem/1(In1)
  If/1 -> If Action Subsystem/Action
  Demux1/1 -> If/1
  Demux/1 -> Compare To Constant/1, Relational Operator1/2
  Demux/2 -> Triggered Subsystem1/1(In1)
  FWNum/1 -> Relational Operator1/1
  TC_FW_ModeSet/1 -> Demux/1
  Relational Operator1/1 -> Logical Operator/2
  Logical Operator/1 -> Triggered Subsystem1/Enable
  Compare To Constant/1 -> Logical Operator/1

== system GS_model/Subsystem2/Subsystem/Actuator/FlyWheel/FwAModel2/FWDataSourceChoice/DelayModel ==
  TC_FW_Delay : Inport
  FW_Cmd_Mode : Inport  Port=2
  FW_Cmd_Spd : Inport  Port=3
  FW_Cmd_T : Inport  Port=4
  Constant3 : Constant
  Sum8 : Sum  Inputs=|++
  delay1 : Subsystem
  delay2 : Subsystem
  delay3 : Subsystem
  Cmd_Mode : Outport
  Cmd_Spd : Outport  Port=2
  Cmd_T : Outport  Port=3
  wires:
  delay3/1(Out1) -> Cmd_Mode/1
  FW_Cmd_Mode/1 -> delay3/2(In2)
  TC_FW_Delay/1 -> Sum8/1
  Constant3/1 -> Sum8/2
  FW_Cmd_Spd/1 -> delay1/2(In2)
  Sum8/1 -> delay3/1(In1), delay2/1(In1), delay1/1(In1)
  delay1/1(Out1) -> Cmd_Spd/1
  FW_Cmd_T/1 -> delay2/2(In2)
  delay2/1(Out1) -> Cmd_T/1

== system GS_model/Subsystem2/Subsystem/Actuator/FlyWheel/FwAModel2/FWMath&ErrModel/Subsystem1 ==
  Fb_FW_T : Inport
  TC_FW_TSet : Inport  Port=2
  FWNum : Inport  Port=3
  TC_FWErr_TOp : Inport  Port=4
  Compare To Constant : simulink/Logic and Bit Operations/Compare To Constant  relop===  const=0  OutDataTypeStr=boolean
  Compare To Constant1 : simulink/Logic and Bit Operations/Compare To Constant  relop===  const=0  OutDataTypeStr=boolean
  Demux : Demux  Outputs=[1;2]
  Demux1 : Demux  Outputs=2
  Demux2 : Demux  Outputs=2
  If : If  IfExpression=u1 == 1
  If Action Subsystem : Subsystem  TreatAsAtomicUnit=on
  If Action Subsystem1 : Subsystem  TreatAsAtomicUnit=on
  Logical Operator : Logic  Operator=OR  AllPortsSameDT=off  OutDataTypeStr=boolean
  Logical Operator1 : Logic  Operator=OR  AllPortsSameDT=off  OutDataTypeStr=boolean
  Merge : Merge
  Relational Operator1 : RelationalOperator  Operator===  OutDataTypeStr=boolean  RndMeth=Simplest
  Relational Operator3 : RelationalOperator  Operator===  OutDataTypeStr=boolean  RndMeth=Simplest
  Sum : Sum  Inputs=|++
  Triggered Subsystem1 : Subsystem  TreatAsAtomicUnit=on
      mask Display: disp('FWChoice')
  Triggered Subsystem2 : Subsystem  TreatAsAtomicUnit=on
      mask Display: disp('FWChoice')
  TM_FW_T : Outport
  wires:
  FWNum/1 -> Relational Operator3/1, Relational Operator1/1
  Compare To Constant1/1 -> Logical Operator1/1
  Relational Operator1/1 -> Logical Operator1/2
  Demux2/1 -> Compare To Constant1/1, Relational Operator1/2
  Logical Operator1/1 -> Triggered Subsystem2/Enable
  Logical Operator/1 -> Triggered Subsystem1/Enable
  Demux/1 -> Relational Operator3/2, Compare To Constant/1
  Relational Operator3/1 -> Logical Operator/2
  Compare To Constant/1 -> Logical Operator/1
  Demux1/1 -> If/1
  If Action Subsystem/1(Out1) -> Merge/1
  Triggered Subsystem1/1(Out1) -> Demux1/1
  Demux/2 -> Triggered Subsystem1/1(In1)
  If/1 -> If Action Subsystem/Action
  TC_FW_TSet/1 -> Demux/1
  Sum/1 -> If Action Subsystem1/1(In1)
  Merge/1 -> TM_FW_T/1
  TC_FWErr_TOp/1 -> Demux2/1
  Demux2/2 -> Triggered Subsystem2/1(In1)
  Triggered Subsystem2/1(Out1) -> Sum/1
  If Action Subsystem1/1(Out1) -> Merge/2
  Demux1/2 -> If Action Subsystem/1(In1)
  If/2 -> If Action Subsystem1/Action
  Fb_FW_T/1 -> Sum/2

== system GS_model/Subsystem2/Subsystem/Actuator/FlyWheel/FwAModel2/FWMath&ErrModel/Subsystem2 ==
  Fb_FW_Spd : Inport
  TC_FW_SpdSet : Inport  Port=2
  FWNum : Inport  Port=3
  TC_FWErr_SpdOp : Inport  Port=4
  Compare To Constant : simulink/Logic and Bit Operations/Compare To Constant  relop===  const=0  OutDataTypeStr=boolean
  Compare To Constant1 : simulink/Logic and Bit Operations/Compare To Constant  relop===  const=0  OutDataTypeStr=boolean
  Demux : Demux  Outputs=[1;2]
  Demux1 : Demux  Outputs=2
  Demux2 : Demux  Outputs=2
  If : If  IfExpression=u1 == 1
  If Action Subsystem : Subsystem  TreatAsAtomicUnit=on
  If Action Subsystem1 : Subsystem  TreatAsAtomicUnit=on
  Logical Operator : Logic  Operator=OR  AllPortsSameDT=off  OutDataTypeStr=boolean
  Logical Operator1 : Logic  Operator=OR  AllPortsSameDT=off  OutDataTypeStr=boolean
  Merge : Merge
  Relational Operator1 : RelationalOperator  Operator===  OutDataTypeStr=boolean  RndMeth=Simplest
  Relational Operator2 : RelationalOperator  Operator===  OutDataTypeStr=boolean  RndMeth=Simplest
  Sum : Sum  Inputs=|++
  Triggered Subsystem1 : Subsystem  TreatAsAtomicUnit=on
      mask Display: disp('FWChoice')
  Triggered Subsystem2 : Subsystem  TreatAsAtomicUnit=on
      mask Display: disp('FWChoice')
  TM_FW_Spd : Outport
  wires:
  Logical Operator1/1 -> Triggered Subsystem2/Enable
  Compare To Constant1/1 -> Logical Operator1/1
  Relational Operator2/1 -> Logical Operator1/2
  Logical Operator/1 -> Triggered Subsystem1/Enable
  Compare To Constant/1 -> Logical Operator/1
  Relational Operator1/1 -> Logical Operator/2
  If/2 -> If Action Subsystem1/Action
  If Action Subsystem/1(Out1) -> Merge/1
  Demux2/1 -> Relational Operator2/2, Compare To Constant1/1
  FWNum/1 -> Relational Operator1/1, Relational Operator2/1
  Triggered Subsystem1/1(Out1) -> Demux1/1
  Fb_FW_Spd/1 -> Sum/2
  Demux/2 -> Triggered Subsystem1/1(In1)
  If Action Subsystem1/1(Out1) -> Merge/2
  Demux1/1 -> If/1
  Demux2/2 -> Triggered Subsystem2/1(In1)
  Demux1/2 -> If Action Subsystem/1(In1)
  Sum/1 -> If Action Subsystem1/1(In1)
  Triggered Subsystem2/1(Out1) -> Sum/1
  TC_FWErr_SpdOp/1 -> Demux2/1
  If/1 -> If Action Subsystem/Action
  Merge/1 -> TM_FW_Spd/1
  Demux/1 -> Relational Operator1/2, Compare To Constant/1
  TC_FW_SpdSet/1 -> Demux/1

== system GS_model/Subsystem2/Subsystem/Actuator/FlyWheel/FwAModel2/FWMath&ErrModel/Subsystem4 ==
  FWNum : Inport
  FW_Mode : Inport  Port=2
  TC_FW_ModeSet : Inport  Port=3
  Compare To Constant : simulink/Logic and Bit Operations/Compare To Constant  relop===  const=0  OutDataTypeStr=boolean
  Demux : Demux  Outputs=[1;2]
  Demux1 : Demux  Outputs=2
  If : If  IfExpression=u1 == 1
  If Action Subsystem : Subsystem  TreatAsAtomicUnit=on
  If Action Subsystem1 : Subsystem  TreatAsAtomicUnit=on
  Logical Operator : Logic  Operator=OR  AllPortsSameDT=off  OutDataTypeStr=boolean
  Merge : Merge
  Relational Operator1 : RelationalOperator  Operator===  OutDataTypeStr=boolean  RndMeth=Simplest
  Triggered Subsystem1 : Subsystem  TreatAsAtomicUnit=on
      mask Display: disp('FWChoice')
  Fb_FW_Mode : Outport
  wires:
  Compare To Constant/1 -> Logical Operator/1
  Logical Operator/1 -> Triggered Subsystem1/Enable
  Relational Operator1/1 -> Logical Operator/2
  TC_FW_ModeSet/1 -> Demux/1
  FWNum/1 -> Relational Operator1/1
  Demux/2 -> Triggered Subsystem1/1(In1)
  Demux/1 -> Relational Operator1/2, Compare To Constant/1
  Demux1/1 -> If/1
  If/1 -> If Action Subsystem/Action
  Demux1/2 -> If Action Subsystem/1(In1)
  Triggered Subsystem1/1(Out1) -> Demux1/1
  If/2 -> If Action Subsystem1/Action
  FW_Mode/1 -> If Action Subsystem1/1(In1)
  If Action Subsystem/1(Out1) -> Merge/1
  If Action Subsystem1/1(Out1) -> Merge/2
  Merge/1 -> Fb_FW_Mode/1

== system GS_model/Subsystem2/Subsystem/Actuator/FlyWheel/FwAModel3/FWDataSourceChoice/DelayModel ==
  TC_FW_Delay : Inport
  FW_Cmd_Mode : Inport  Port=2
  FW_Cmd_Spd : Inport  Port=3
  FW_Cmd_T : Inport  Port=4
  Constant3 : Constant
  Sum8 : Sum  Inputs=|++
  delay1 : Subsystem
  delay2 : Subsystem
  delay3 : Subsystem
  Cmd_Mode : Outport
  Cmd_Spd : Outport  Port=2
  Cmd_T : Outport  Port=3
  wires:
  delay2/1(Out1) -> Cmd_T/1
  FW_Cmd_T/1 -> delay2/2(In2)
  delay1/1(Out1) -> Cmd_Spd/1
  Sum8/1 -> delay1/1(In1), delay2/1(In1), delay3/1(In1)
  FW_Cmd_Spd/1 -> delay1/2(In2)
  Constant3/1 -> Sum8/2
  TC_FW_Delay/1 -> Sum8/1
  FW_Cmd_Mode/1 -> delay3/2(In2)
  delay3/1(Out1) -> Cmd_Mode/1

== system GS_model/Subsystem2/Subsystem/Actuator/FlyWheel/FwAModel3/FWMath&ErrModel/Subsystem1 ==
  Fb_FW_T : Inport
  TC_FW_TSet : Inport  Port=2
  FWNum : Inport  Port=3
  TC_FWErr_TOp : Inport  Port=4
  Compare To Constant : simulink/Logic and Bit Operations/Compare To Constant  relop===  const=0  OutDataTypeStr=boolean
  Compare To Constant1 : simulink/Logic and Bit Operations/Compare To Constant  relop===  const=0  OutDataTypeStr=boolean
  Demux : Demux  Outputs=[1;2]
  Demux1 : Demux  Outputs=2
  Demux2 : Demux  Outputs=2
  If : If  IfExpression=u1 == 1
  If Action Subsystem : Subsystem  TreatAsAtomicUnit=on
  If Action Subsystem1 : Subsystem  TreatAsAtomicUnit=on
  Logical Operator : Logic  Operator=OR  AllPortsSameDT=off  OutDataTypeStr=boolean
  Logical Operator1 : Logic  Operator=OR  AllPortsSameDT=off  OutDataTypeStr=boolean
  Merge : Merge
  Relational Operator1 : RelationalOperator  Operator===  OutDataTypeStr=boolean  RndMeth=Simplest
  Relational Operator3 : RelationalOperator  Operator===  OutDataTypeStr=boolean  RndMeth=Simplest
  Sum : Sum  Inputs=|++
  Triggered Subsystem1 : Subsystem  TreatAsAtomicUnit=on
      mask Display: disp('FWChoice')
  Triggered Subsystem2 : Subsystem  TreatAsAtomicUnit=on
      mask Display: disp('FWChoice')
  TM_FW_T : Outport
  wires:
  Fb_FW_T/1 -> Sum/2
  If/2 -> If Action Subsystem1/Action
  Demux1/2 -> If Action Subsystem/1(In1)
  If Action Subsystem1/1(Out1) -> Merge/2
  Triggered Subsystem2/1(Out1) -> Sum/1
  Demux2/2 -> Triggered Subsystem2/1(In1)
  TC_FWErr_TOp/1 -> Demux2/1
  Merge/1 -> TM_FW_T/1
  Sum/1 -> If Action Subsystem1/1(In1)
  TC_FW_TSet/1 -> Demux/1
  If/1 -> If Action Subsystem/Action
  Demux/2 -> Triggered Subsystem1/1(In1)
  Triggered Subsystem1/1(Out1) -> Demux1/1
  If Action Subsystem/1(Out1) -> Merge/1
  Demux1/1 -> If/1
  Compare To Constant/1 -> Logical Operator/1
  Relational Operator3/1 -> Logical Operator/2
  Demux/1 -> Compare To Constant/1, Relational Operator3/2
  Logical Operator/1 -> Triggered Subsystem1/Enable
  Logical Operator1/1 -> Triggered Subsystem2/Enable
  Demux2/1 -> Relational Operator1/2, Compare To Constant1/1
  Relational Operator1/1 -> Logical Operator1/2
  Compare To Constant1/1 -> Logical Operator1/1
  FWNum/1 -> Relational Operator1/1, Relational Operator3/1

== system GS_model/Subsystem2/Subsystem/Actuator/FlyWheel/FwAModel3/FWMath&ErrModel/Subsystem2 ==
  Fb_FW_Spd : Inport
  TC_FW_SpdSet : Inport  Port=2
  FWNum : Inport  Port=3
  TC_FWErr_SpdOp : Inport  Port=4
  Compare To Constant : simulink/Logic and Bit Operations/Compare To Constant  relop===  const=0  OutDataTypeStr=boolean
  Compare To Constant1 : simulink/Logic and Bit Operations/Compare To Constant  relop===  const=0  OutDataTypeStr=boolean
  Demux : Demux  Outputs=[1;2]
  Demux1 : Demux  Outputs=2
  Demux2 : Demux  Outputs=2
  If : If  IfExpression=u1 == 1
  If Action Subsystem : Subsystem  TreatAsAtomicUnit=on
  If Action Subsystem1 : Subsystem  TreatAsAtomicUnit=on
  Logical Operator : Logic  Operator=OR  AllPortsSameDT=off  OutDataTypeStr=boolean
  Logical Operator1 : Logic  Operator=OR  AllPortsSameDT=off  OutDataTypeStr=boolean
  Merge : Merge
  Relational Operator1 : RelationalOperator  Operator===  OutDataTypeStr=boolean  RndMeth=Simplest
  Relational Operator2 : RelationalOperator  Operator===  OutDataTypeStr=boolean  RndMeth=Simplest
  Sum : Sum  Inputs=|++
  Triggered Subsystem1 : Subsystem  TreatAsAtomicUnit=on
      mask Display: disp('FWChoice')
  Triggered Subsystem2 : Subsystem  TreatAsAtomicUnit=on
      mask Display: disp('FWChoice')
  TM_FW_Spd : Outport
  wires:
  TC_FW_SpdSet/1 -> Demux/1
  Demux/1 -> Compare To Constant/1, Relational Operator1/2
  Merge/1 -> TM_FW_Spd/1
  If/1 -> If Action Subsystem/Action
  TC_FWErr_SpdOp/1 -> Demux2/1
  Triggered Subsystem2/1(Out1) -> Sum/1
  Sum/1 -> If Action Subsystem1/1(In1)
  Demux1/2 -> If Action Subsystem/1(In1)
  Demux2/2 -> Triggered Subsystem2/1(In1)
  Demux1/1 -> If/1
  If Action Subsystem1/1(Out1) -> Merge/2
  Demux/2 -> Triggered Subsystem1/1(In1)
  Fb_FW_Spd/1 -> Sum/2
  Triggered Subsystem1/1(Out1) -> Demux1/1
  FWNum/1 -> Relational Operator2/1, Relational Operator1/1
  Demux2/1 -> Compare To Constant1/1, Relational Operator2/2
  If Action Subsystem/1(Out1) -> Merge/1
  If/2 -> If Action Subsystem1/Action
  Relational Operator1/1 -> Logical Operator/2
  Compare To Constant/1 -> Logical Operator/1
  Logical Operator/1 -> Triggered Subsystem1/Enable
  Relational Operator2/1 -> Logical Operator1/2
  Compare To Constant1/1 -> Logical Operator1/1
  Logical Operator1/1 -> Triggered Subsystem2/Enable

== system GS_model/Subsystem2/Subsystem/Actuator/FlyWheel/FwAModel3/FWMath&ErrModel/Subsystem4 ==
  FWNum : Inport
  FW_Mode : Inport  Port=2
  TC_FW_ModeSet : Inport  Port=3
  Compare To Constant : simulink/Logic and Bit Operations/Compare To Constant  relop===  const=0  OutDataTypeStr=boolean
  Demux : Demux  Outputs=[1;2]
  Demux1 : Demux  Outputs=2
  If : If  IfExpression=u1 == 1
  If Action Subsystem : Subsystem  TreatAsAtomicUnit=on
  If Action Subsystem1 : Subsystem  TreatAsAtomicUnit=on
  Logical Operator : Logic  Operator=OR  AllPortsSameDT=off  OutDataTypeStr=boolean
  Merge : Merge
  Relational Operator1 : RelationalOperator  Operator===  OutDataTypeStr=boolean  RndMeth=Simplest
  Triggered Subsystem1 : Subsystem  TreatAsAtomicUnit=on
      mask Display: disp('FWChoice')
  Fb_FW_Mode : Outport
  wires:
  Merge/1 -> Fb_FW_Mode/1
  If Action Subsystem1/1(Out1) -> Merge/2
  If Action Subsystem/1(Out1) -> Merge/1
  FW_Mode/1 -> If Action Subsystem1/1(In1)
  If/2 -> If Action Subsystem1/Action
  Triggered Subsystem1/1(Out1) -> Demux1/1
  Demux1/2 -> If Action Subsystem/1(In1)
  If/1 -> If Action Subsystem/Action
  Demux1/1 -> If/1
  Demux/1 -> Compare To Constant/1, Relational Operator1/2
  Demux/2 -> Triggered Subsystem1/1(In1)
  FWNum/1 -> Relational Operator1/1
  TC_FW_ModeSet/1 -> Demux/1
  Relational Operator1/1 -> Logical Operator/2
  Logical Operator/1 -> Triggered Subsystem1/Enable
  Compare To Constant/1 -> Logical Operator/1

== system GS_model/Subsystem2/Subsystem/Actuator/FlyWheel/FwAModel4/FWDataSourceChoice/DelayModel ==
  TC_FW_Delay : Inport
  FW_Cmd_Mode : Inport  Port=2
  FW_Cmd_Spd : Inport  Port=3
  FW_Cmd_T : Inport  Port=4
  Constant3 : Constant
  Sum8 : Sum  Inputs=|++
  delay1 : Subsystem
  delay2 : Subsystem
  delay3 : Subsystem
  Cmd_Mode : Outport
  Cmd_Spd : Outport  Port=2
  Cmd_T : Outport  Port=3
  wires:
  delay3/1(Out1) -> Cmd_Mode/1
  FW_Cmd_Mode/1 -> delay3/2(In2)
  TC_FW_Delay/1 -> Sum8/1
  Constant3/1 -> Sum8/2
  FW_Cmd_Spd/1 -> delay1/2(In2)
  Sum8/1 -> delay3/1(In1), delay2/1(In1), delay1/1(In1)
  delay1/1(Out1) -> Cmd_Spd/1
  FW_Cmd_T/1 -> delay2/2(In2)
  delay2/1(Out1) -> Cmd_T/1
